simulink model "control_system"  (R2021a)
settings: Solver=VariableStepAuto  StartTime=0.0  StopTime=10.0  MaxStep=1/10000  RelTol=1e-3
values from neighbouring files (symbols this model uses):
  A = 8    [laplace_transform.m]
  B = 0    [laplace_transform.m]
  C = 7    [laplace_transform.m]
  D = 1    [laplace_transform.m]
  F = 6    [laplace_transform.m]
  G = 10    [laplace_transform.m]
settings Model: Creator=Abdelrahman  LastModifiedBy=User
settings SolverCC: AlgebraicLoopSolver=TrustRegion
settings DebuggingCC: SFMachineParentedDataDiag=warning
settings SFSimCC: CustomCodeUndefinedFunction=UseInterfaceOnly

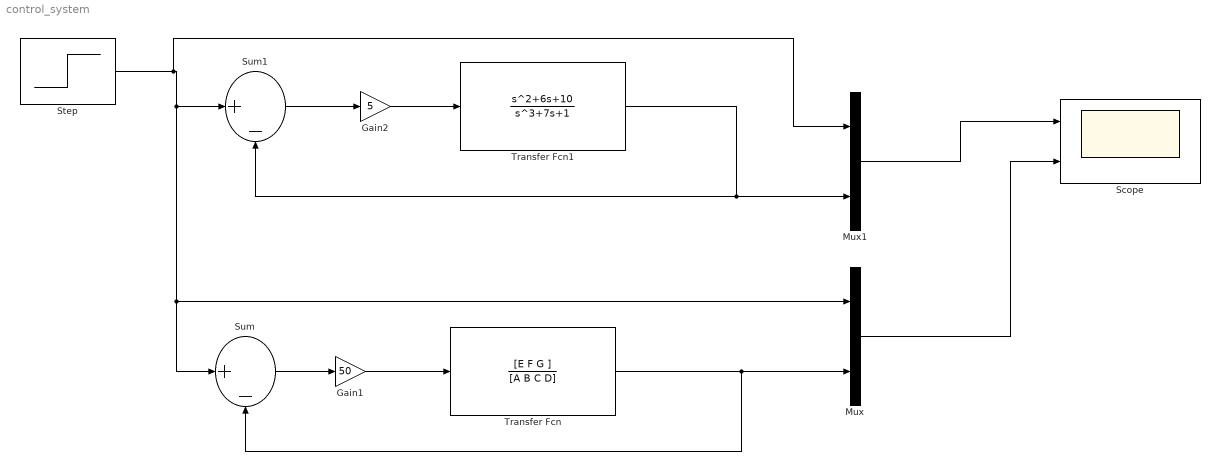
== system control_system ==
  Gain1 : Gain  Gain=50
  Gain2 : Gain  Gain=5
  Mux : Mux  Inputs=2
  Mux1 : Mux  Inputs=2
  Scope : Scope  NumInputPorts=2
  Step : Step  SampleTime=0
  Sum : Sum  Inputs=|+-
  Sum1 : Sum  Inputs=|+-
  Transfer Fcn : TransferFcn  Numerator=[E F G ]  Denominator=[A B C D]
  Transfer Fcn1 : TransferFcn  Numerator=[1 6 10]  Denominator=[1 0 7 1]
  wires:
  Gain2/1 -> Transfer Fcn1/1
  Sum1/1 -> Gain2/1
  Transfer Fcn1/1 -> Mux1/2, Sum1/2
  Transfer Fcn/1 -> Sum/2, Mux/2
  Mux/1 -> Scope/2
  Step/1 -> Mux1/1, Mux/1, Sum/1, Sum1/1
  Mux1/1 -> Scope/1
  Sum/1 -> Gain1/1
  Gain1/1 -> Transfer Fcn/1
